simulink model "OceanForce"  (R2018b)
settings: Solver=VariableStepAuto  StartTime=0.0  StopTime=tsim  RelTol=1e-3
undefined symbols (not defined in the file or in its folder): Cd, Cm, D, gamma, H, h, k, kk, Tperiod
settings Model: Creator=Erin B  LastModifiedBy=Erin B

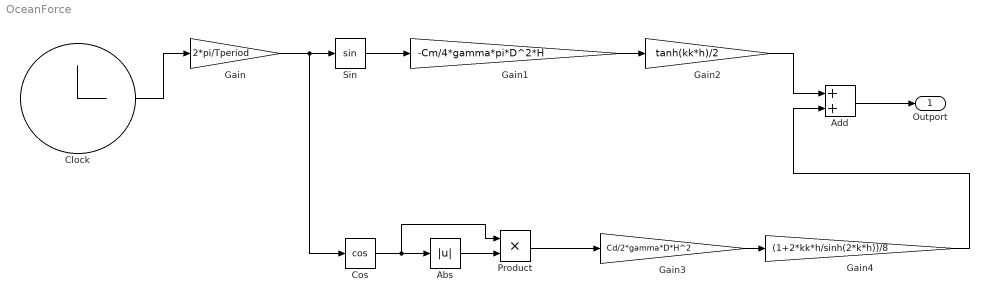
== system OceanForce ==
  Abs : Abs
  Add : Sum
  Clock : Clock
  Cos : Trigonometry  Operator=cos
  Gain : Gain  Gain=2*pi/Tperiod
  Gain1 : Gain  Gain=-Cm/4*gamma*pi*D^2*H
  Gain2 : Gain  Gain=tanh(kk*h)/2
  Gain3 : Gain  Gain=Cd/2*gamma*D*H^2
  Gain4 : Gain  Gain=(1+2*kk*h/sinh(2*k*h))/8
  Product : Product
  Sin : Trigonometry
  Outport : Outport
  wires:
  Clock/1 -> Gain/1
  Gain/1 -> Cos/1, Sin/1
  Sin/1 -> Gain1/1
  Gain1/1 -> Gain2/1
  Add/1 -> Outport/1
  Gain2/1 -> Add/1
  Cos/1 -> Product/1, Abs/1
  Abs/1 -> Product/2
  Product/1 -> Gain3/1
  Gain3/1 -> Gain4/1
  Gain4/1 -> Add/2
